simulink model "gm_DUALportRAMinterface_v3_vnl"  (R2024a)
settings: Solver=FixedStepDiscrete  StartTime=0.0  StopTime=20  RelTol=1e-3
undefined symbols (not defined in the file or in its folder): magnitude, Ts
libraries: hdlsllib x419, hdlmdlgenlib x103, embmathops x12, simulink x5, dsphdlxfrm2 x2
(part 7 of 11)

== system gm_DUALportRAMinterface_v3_vnl/PL/integration_block1/GA_main/coefficent_array/individual4 ==
  reg_in : Inport  OutDataTypeStr=fixdt(1, 33, 15)  PortDimensions=1  SampleTime=3.00000003e-08
  reg_in1 : Inport  Port=2  OutDataTypeStr=fixdt(1, 33, 15)  PortDimensions=1  SampleTime=3.00000003e-08
  reg_in2 : Inport  Port=3  OutDataTypeStr=fixdt(1, 33, 15)  PortDimensions=1  SampleTime=3.00000003e-08
  reg_in3 : Inport  Port=4  OutDataTypeStr=fixdt(1, 33, 15)  PortDimensions=1  SampleTime=3.00000003e-08
  reg_in4 : Inport  Port=5  OutDataTypeStr=fixdt(1, 33, 15)  PortDimensions=1  SampleTime=3.00000003e-08
  reg_in5 : Inport  Port=6  OutDataTypeStr=fixdt(1, 33, 15)  PortDimensions=1  SampleTime=3.00000003e-08
  reg_in6 : Inport  Port=7  OutDataTypeStr=fixdt(1, 33, 15)  PortDimensions=1  SampleTime=3.00000003e-08
  enable : Inport  Port=8  OutDataTypeStr=boolean  PortDimensions=1  SampleTime=3.00000003e-08
  Subsystem : Subsystem
  Subsystem1 : Subsystem
  Subsystem2 : Subsystem
  Subsystem3 : Subsystem
  Subsystem4 : Subsystem
  Subsystem5 : Subsystem
  Subsystem6 : Subsystem
  score : Outport  SampleTime=3.00000003e-08
  a2 : Outport  Port=2  SampleTime=3.00000003e-08
  a3 : Outport  Port=3  SampleTime=3.00000003e-08
  a4 : Outport  Port=4  SampleTime=3.00000003e-08
  b2 : Outport  Port=5  SampleTime=3.00000003e-08
  b3 : Outport  Port=6  SampleTime=3.00000003e-08
  b4 : Outport  Port=7  SampleTime=3.00000003e-08
  wires:
  Subsystem6/1(reg_out) -> b4/1
  Subsystem5/1(reg_out) -> b3/1
  Subsystem4/1(reg_out) -> b2/1
  Subsystem3/1(reg_out) -> a4/1
  Subsystem2/1(reg_out) -> a3/1
  Subsystem1/1(reg_out) -> a2/1
  Subsystem/1(reg_out) -> score/1
  enable/1 -> Subsystem3/2(enable), Subsystem4/2(enable), Subsystem5/2(enable), Subsystem6/2(enable), Subsystem2/2(enable), Subsystem1/2(enable), Subsystem/2(enable)
  reg_in6/1 -> Subsystem6/1(reg_in)
  reg_in5/1 -> Subsystem5/1(reg_in)
  reg_in4/1 -> Subsystem4/1(reg_in)
  reg_in3/1 -> Subsystem3/1(reg_in)
  reg_in2/1 -> Subsystem2/1(reg_in)
  reg_in1/1 -> Subsystem1/1(reg_in)
  reg_in/1 -> Subsystem/1(reg_in)

== system gm_DUALportRAMinterface_v3_vnl/PL/integration_block1/GA_main/coefficent_array/output_selector ==
  chose_port : Inport  OutDataTypeStr=fixdt(0, 4, 0)  PortDimensions=1  SampleTime=3.00000003e-08
  In2 : Inport  Port=2  OutDataTypeStr=fixdt(1, 33, 15)  PortDimensions=[7]  SampleTime=3.00000003e-08
  In3 : Inport  Port=3  OutDataTypeStr=fixdt(1, 33, 15)  PortDimensions=[7]  SampleTime=3.00000003e-08
  In4 : Inport  Port=4  OutDataTypeStr=fixdt(1, 33, 15)  PortDimensions=[7]  SampleTime=3.00000003e-08
  In5 : Inport  Port=5  OutDataTypeStr=fixdt(1, 33, 15)  PortDimensions=[7]  SampleTime=3.00000003e-08
  Multiport Switch : MultiPortSwitch  Inputs=4  OutDataTypeStr=fixdt(1, 33, 15)  SaturateOnIntegerOverflow=off  InputSameDT=off
  Switch : Switch  Criteria=u2 > Threshold  OutDataTypeStr=fixdt(1, 33, 15)  SaturateOnIntegerOverflow=off  InputSameDT=off
  Switch1 : Switch  Criteria=u2 > Threshold  OutDataTypeStr=fixdt(0, 4, 0)  SaturateOnIntegerOverflow=off  InputSameDT=off
  default_value : Constant  OutDataTypeStr=fixdt(0,4,0)  SampleTime=Ts
  ensure_correct_output : Constant  Value=0  OutDataTypeStr=fixdt(0,1,0)  SampleTime=Ts
  Out1 : Outport  SampleTime=3.00000003e-08
  wires:
  ensure_correct_output/1 -> Switch/3
  default_value/1 -> Switch1/3
  Switch1/1 -> Multiport Switch/1
  Switch/1 -> Out1/1
  Multiport Switch/1 -> Switch/1
  In5/1 -> Multiport Switch/5
  In4/1 -> Multiport Switch/4
  In3/1 -> Multiport Switch/3
  In2/1 -> Multiport Switch/2
  chose_port/1 -> Switch/2, Switch1/1, Switch1/2

== system gm_DUALportRAMinterface_v3_vnl/PL/integration_block1/GA_main/coefficent_array/swap_counter ==
  In1 : Inport  OutDataTypeStr=boolean  PortDimensions=1  SampleTime=3.00000003e-08
  In2 : Inport  Port=2  OutDataTypeStr=boolean  PortDimensions=1  SampleTime=3.00000003e-08
  Add : Sum  OutDataTypeStr=fixdt(0,4,0)  AccumDataTypeStr=fixdt(0,4,0)
  Constant18 : Constant  OutDataTypeStr=fixdt(0,4,0)  SampleTime=Ts
  Constant19 : Constant  Value=0  OutDataTypeStr=fixdt(0,4,0)  SampleTime=Ts
  Constant20 : Constant  Value=0  OutDataTypeStr=fixdt(0,4,0)  SampleTime=Ts
  Delay : Delay  DelayLength=1  InitialCondition=0  SampleTime=Ts
  Switch : Switch  Criteria=u2 > Threshold  OutDataTypeStr=fixdt(0,4,0)  SaturateOnIntegerOverflow=off  InputSameDT=off
  Switch8 : Switch  Criteria=u2 > Threshold  OutDataTypeStr=fixdt(0,4,0)  SaturateOnIntegerOverflow=off  InputSameDT=off
  Out1 : Outport  SampleTime=3.00000003e-08
  wires:
  Switch8/1 -> Add/2
  Add/1 -> Delay/1
  Switch/1 -> Add/1
  In2/1 -> Switch8/2
  Constant20/1 -> Switch8/1
  Delay/1 -> Switch8/3, Out1/1
  Constant19/1 -> Switch/3
  Constant18/1 -> Switch/1
  In1/1 -> Switch/2

== system gm_DUALportRAMinterface_v3_vnl/PL/integration_block1/GA_main/coefficent_array/swap_counter1 ==
  In1 : Inport  OutDataTypeStr=boolean  PortDimensions=1  SampleTime=3.00000003e-08
  In2 : Inport  Port=2  OutDataTypeStr=boolean  PortDimensions=1  SampleTime=3.00000003e-08
  Add : Sum  OutDataTypeStr=fixdt(0,4,0)  AccumDataTypeStr=fixdt(0,4,0)
  Constant18 : Constant  OutDataTypeStr=fixdt(0,4,0)  SampleTime=Ts
  Constant19 : Constant  Value=0  OutDataTypeStr=fixdt(0,4,0)  SampleTime=Ts
  Constant20 : Constant  OutDataTypeStr=fixdt(0,4,0)  SampleTime=Ts
  Delay : Delay  DelayLength=1  InitialCondition=0  SampleTime=Ts
  Switch : Switch  Criteria=u2 > Threshold  OutDataTypeStr=fixdt(0,4,0)  SaturateOnIntegerOverflow=off  InputSameDT=off
  Switch8 : Switch  Criteria=u2 > Threshold  OutDataTypeStr=fixdt(0,4,0)  SaturateOnIntegerOverflow=off  InputSameDT=off
  Out1 : Outport  SampleTime=3.00000003e-08
  wires:
  Switch8/1 -> Add/2
  Add/1 -> Delay/1
  Switch/1 -> Add/1
  In2/1 -> Switch8/2
  Constant20/1 -> Switch8/1
  Delay/1 -> Switch8/3, Out1/1
  Constant19/1 -> Switch/3
  Constant18/1 -> Switch/1
  In1/1 -> Switch/2

== system gm_DUALportRAMinterface_v3_vnl/PL/integration_block1/GA_main/coefficent_array1/Chart ==
  index : Inport  OutDataTypeStr=fixdt(0, 4, 0)  PortDimensions=1  SampleTime=3.00000003e-08
  start_sort : Inport  Port=2  OutDataTypeStr=boolean  PortDimensions=1  SampleTime=3.00000003e-08
  swaps_in : Inport  Port=3  OutDataTypeStr=fixdt(0, 4, 0)  PortDimensions=1  SampleTime=3.00000003e-08
  swap_signal : Inport  Port=4  OutDataTypeStr=boolean  PortDimensions=1  SampleTime=3.00000003e-08
  Chart : Stateflow chart  TreatAsAtomicUnit=on
      settings: PortSchema="{\"entries\":[{\"content\":{\"sides\":[{\"content\":{\"connectorIds\":[\"In1\",\"In4\",\"In3\"]},\"type\":\"ConnectorPlacement.EquallySpacedRectSide\",\"uuid\":\"bd2dafac-a5a9-4836-b8bd-cefb36fb6626\"},{\"content\":{\"connectorIds\":[\"Out1\",\"Out2\",\"Out3\",\"Out4\",\"Out5\",\"Out6\"],\"side\":\"RIGHT\"},\"type\":\"ConnectorPlacement.EquallySpacedRectSide\",\"uuid\":\"b2eb894e-8d56-4038-acbe-51c43d919a15\"},{\"content\":{\"connectorIds\":[\"In2\"],\"side\":\"TOP\"},\"type\":\"ConnectorPlacement.EquallySpacedRectSide\",\"uuid\":\"645ecb99-1eca-4a2d-8e44-d34ac75e3d1a\"}]},\"type\":\"ConnectorPlacement.EquallySpacedConnector\",\"uuid\":\"63f53eab-c5ec-482c-b992-d953653b0c27\"}],\"packageUris\":[\"http://schema.mathworks.com/mf0/Connector/R2020b\"],\"version\":\"1.0\"}"
  index_increment : Outport  SampleTime=3.00000003e-08
  index_reset : Outport  Port=2  SampleTime=3.00000003e-08
  sort_done : Outport  Port=3  SampleTime=3.00000003e-08
  commit_swap : Outport  Port=4  SampleTime=3.00000003e-08
  swaps_increment : Outport  Port=5  SampleTime=3.00000003e-08
  reset_swaps : Outport  Port=6  SampleTime=3.00000003e-08
  wires:
  Chart/6(reset_swaps) -> reset_swaps/1
  Chart/5(swaps_increment) -> swaps_increment/1
  Chart/4(commit_swap) -> commit_swap/1
  Chart/3(sort_done) -> sort_done/1
  Chart/2(index_reset) -> index_reset/1
  Chart/1(index_increment) -> index_increment/1
  swap_signal/1 -> Chart/4(swap_signal)
  swaps_in/1 -> Chart/3(swaps_in)
  start_sort/1 -> Chart/2(start_sort)
  index/1 -> Chart/1(index)

== system gm_DUALportRAMinterface_v3_vnl/PL/integration_block1/GA_main/coefficent_array1/individual1 ==
  reg_in : Inport  OutDataTypeStr=fixdt(1, 33, 15)  PortDimensions=1  SampleTime=3.00000003e-08
  reg_in1 : Inport  Port=2  OutDataTypeStr=fixdt(1, 33, 15)  PortDimensions=1  SampleTime=3.00000003e-08
  reg_in2 : Inport  Port=3  OutDataTypeStr=fixdt(1, 33, 15)  PortDimensions=1  SampleTime=3.00000003e-08
  reg_in3 : Inport  Port=4  OutDataTypeStr=fixdt(1, 33, 15)  PortDimensions=1  SampleTime=3.00000003e-08
  reg_in4 : Inport  Port=5  OutDataTypeStr=fixdt(1, 33, 15)  PortDimensions=1  SampleTime=3.00000003e-08
  reg_in5 : Inport  Port=6  OutDataTypeStr=fixdt(1, 33, 15)  PortDimensions=1  SampleTime=3.00000003e-08
  reg_in6 : Inport  Port=7  OutDataTypeStr=fixdt(1, 33, 15)  PortDimensions=1  SampleTime=3.00000003e-08
  enable : Inport  Port=8  OutDataTypeStr=boolean  PortDimensions=1  SampleTime=3.00000003e-08
  Subsystem : Subsystem
  Subsystem1 : Subsystem
  Subsystem2 : Subsystem
  Subsystem3 : Subsystem
  Subsystem4 : Subsystem
  Subsystem5 : Subsystem
  Subsystem6 : Subsystem
  score : Outport  SampleTime=3.00000003e-08
  a2 : Outport  Port=2  SampleTime=3.00000003e-08
  a3 : Outport  Port=3  SampleTime=3.00000003e-08
  a4 : Outport  Port=4  SampleTime=3.00000003e-08
  b2 : Outport  Port=5  SampleTime=3.00000003e-08
  b3 : Outport  Port=6  SampleTime=3.00000003e-08
  b4 : Outport  Port=7  SampleTime=3.00000003e-08
  wires:
  Subsystem6/1(reg_out) -> b4/1
  Subsystem5/1(reg_out) -> b3/1
  Subsystem4/1(reg_out) -> b2/1
  Subsystem3/1(reg_out) -> a4/1
  Subsystem2/1(reg_out) -> a3/1
  Subsystem1/1(reg_out) -> a2/1
  Subsystem/1(reg_out) -> score/1
  enable/1 -> Subsystem3/2(enable), Subsystem4/2(enable), Subsystem5/2(enable), Subsystem6/2(enable), Subsystem2/2(enable), Subsystem1/2(enable), Subsystem/2(enable)
  reg_in6/1 -> Subsystem6/1(reg_in)
  reg_in5/1 -> Subsystem5/1(reg_in)
  reg_in4/1 -> Subsystem4/1(reg_in)
  reg_in3/1 -> Subsystem3/1(reg_in)
  reg_in2/1 -> Subsystem2/1(reg_in)
  reg_in1/1 -> Subsystem1/1(reg_in)
  reg_in/1 -> Subsystem/1(reg_in)

== system gm_DUALportRAMinterface_v3_vnl/PL/integration_block1/GA_main/coefficent_array1/individual2 ==
  reg_in : Inport  OutDataTypeStr=fixdt(1, 33, 15)  PortDimensions=1  SampleTime=3.00000003e-08
  reg_in1 : Inport  Port=2  OutDataTypeStr=fixdt(1, 33, 15)  PortDimensions=1  SampleTime=3.00000003e-08
  reg_in2 : Inport  Port=3  OutDataTypeStr=fixdt(1, 33, 15)  PortDimensions=1  SampleTime=3.00000003e-08
  reg_in3 : Inport  Port=4  OutDataTypeStr=fixdt(1, 33, 15)  PortDimensions=1  SampleTime=3.00000003e-08
  reg_in4 : Inport  Port=5  OutDataTypeStr=fixdt(1, 33, 15)  PortDimensions=1  SampleTime=3.00000003e-08
  reg_in5 : Inport  Port=6  OutDataTypeStr=fixdt(1, 33, 15)  PortDimensions=1  SampleTime=3.00000003e-08
  reg_in6 : Inport  Port=7  OutDataTypeStr=fixdt(1, 33, 15)  PortDimensions=1  SampleTime=3.00000003e-08
  enable : Inport  Port=8  OutDataTypeStr=boolean  PortDimensions=1  SampleTime=3.00000003e-08
  Subsystem : Subsystem
  Subsystem1 : Subsystem
  Subsystem2 : Subsystem
  Subsystem3 : Subsystem
  Subsystem4 : Subsystem
  Subsystem5 : Subsystem
  Subsystem6 : Subsystem
  score : Outport  SampleTime=3.00000003e-08
  a2 : Outport  Port=2  SampleTime=3.00000003e-08
  a3 : Outport  Port=3  SampleTime=3.00000003e-08
  a4 : Outport  Port=4  SampleTime=3.00000003e-08
  b2 : Outport  Port=5  SampleTime=3.00000003e-08
  b3 : Outport  Port=6  SampleTime=3.00000003e-08
  b4 : Outport  Port=7  SampleTime=3.00000003e-08
  wires:
  Subsystem6/1(reg_out) -> b4/1
  Subsystem5/1(reg_out) -> b3/1
  Subsystem4/1(reg_out) -> b2/1
  Subsystem3/1(reg_out) -> a4/1
  Subsystem2/1(reg_out) -> a3/1
  Subsystem1/1(reg_out) -> a2/1
  Subsystem/1(reg_out) -> score/1
  enable/1 -> Subsystem/2(enable), Subsystem1/2(enable), Subsystem2/2(enable), Subsystem6/2(enable), Subsystem5/2(enable), Subsystem4/2(enable), Subsystem3/2(enable)
  reg_in6/1 -> Subsystem6/1(reg_in)
  reg_in5/1 -> Subsystem5/1(reg_in)
  reg_in4/1 -> Subsystem4/1(reg_in)
  reg_in3/1 -> Subsystem3/1(reg_in)
  reg_in2/1 -> Subsystem2/1(reg_in)
  reg_in1/1 -> Subsystem1/1(reg_in)
  reg_in/1 -> Subsystem/1(reg_in)

== system gm_DUALportRAMinterface_v3_vnl/PL/integration_block1/GA_main/coefficent_array1/individual3 ==
  reg_in : Inport  OutDataTypeStr=fixdt(1, 33, 15)  PortDimensions=1  SampleTime=3.00000003e-08
  reg_in1 : Inport  Port=2  OutDataTypeStr=fixdt(1, 33, 15)  PortDimensions=1  SampleTime=3.00000003e-08
  reg_in2 : Inport  Port=3  OutDataTypeStr=fixdt(1, 33, 15)  PortDimensions=1  SampleTime=3.00000003e-08
  reg_in3 : Inport  Port=4  OutDataTypeStr=fixdt(1, 33, 15)  PortDimensions=1  SampleTime=3.00000003e-08
  reg_in4 : Inport  Port=5  OutDataTypeStr=fixdt(1, 33, 15)  PortDimensions=1  SampleTime=3.00000003e-08
  reg_in5 : Inport  Port=6  OutDataTypeStr=fixdt(1, 33, 15)  PortDimensions=1  SampleTime=3.00000003e-08
  reg_in6 : Inport  Port=7  OutDataTypeStr=fixdt(1, 33, 15)  PortDimensions=1  SampleTime=3.00000003e-08
  enable : Inport  Port=8  OutDataTypeStr=boolean  PortDimensions=1  SampleTime=3.00000003e-08
  Subsystem : Subsystem
  Subsystem1 : Subsystem
  Subsystem2 : Subsystem
  Subsystem3 : Subsystem
  Subsystem4 : Subsystem
  Subsystem5 : Subsystem
  Subsystem6 : Subsystem
  score : Outport  SampleTime=3.00000003e-08
  a2 : Outport  Port=2  SampleTime=3.00000003e-08
  a3 : Outport  Port=3  SampleTime=3.00000003e-08
  a4 : Outport  Port=4  SampleTime=3.00000003e-08
  b2 : Outport  Port=5  SampleTime=3.00000003e-08
  b3 : Outport  Port=6  SampleTime=3.00000003e-08
  b4 : Outport  Port=7  SampleTime=3.00000003e-08
  wires:
  Subsystem6/1(reg_out) -> b4/1
  Subsystem5/1(reg_out) -> b3/1
  Subsystem4/1(reg_out) -> b2/1
  Subsystem3/1(reg_out) -> a4/1
  Subsystem2/1(reg_out) -> a3/1
  Subsystem1/1(reg_out) -> a2/1
  Subsystem/1(reg_out) -> score/1
  enable/1 -> Subsystem3/2(enable), Subsystem4/2(enable), Subsystem5/2(enable), Subsystem6/2(enable), Subsystem2/2(enable), Subsystem1/2(enable), Subsystem/2(enable)
  reg_in6/1 -> Subsystem6/1(reg_in)
  reg_in5/1 -> Subsystem5/1(reg_in)
  reg_in4/1 -> Subsystem4/1(reg_in)
  reg_in3/1 -> Subsystem3/1(reg_in)
  reg_in2/1 -> Subsystem2/1(reg_in)
  reg_in1/1 -> Subsystem1/1(reg_in)
  reg_in/1 -> Subsystem/1(reg_in)

== system gm_DUALportRAMinterface_v3_vnl/PL/integration_block1/GA_main/coefficent_array1/individual4 ==
  reg_in : Inport  OutDataTypeStr=fixdt(1, 33, 15)  PortDimensions=1  SampleTime=3.00000003e-08
  reg_in1 : Inport  Port=2  OutDataTypeStr=fixdt(1, 33, 15)  PortDimensions=1  SampleTime=3.00000003e-08
  reg_in2 : Inport  Port=3  OutDataTypeStr=fixdt(1, 33, 15)  PortDimensions=1  SampleTime=3.00000003e-08
  reg_in3 : Inport  Port=4  OutDataTypeStr=fixdt(1, 33, 15)  PortDimensions=1  SampleTime=3.00000003e-08
  reg_in4 : Inport  Port=5  OutDataTypeStr=fixdt(1, 33, 15)  PortDimensions=1  SampleTime=3.00000003e-08
  reg_in5 : Inport  Port=6  OutDataTypeStr=fixdt(1, 33, 15)  PortDimensions=1  SampleTime=3.00000003e-08
  reg_in6 : Inport  Port=7  OutDataTypeStr=fixdt(1, 33, 15)  PortDimensions=1  SampleTime=3.00000003e-08
  enable : Inport  Port=8  OutDataTypeStr=boolean  PortDimensions=1  SampleTime=3.00000003e-08
  Subsystem : Subsystem
  Subsystem1 : Subsystem
  Subsystem2 : Subsystem
  Subsystem3 : Subsystem
  Subsystem4 : Subsystem
  Subsystem5 : Subsystem
  Subsystem6 : Subsystem
  score : Outport  SampleTime=3.00000003e-08
  a2 : Outport  Port=2  SampleTime=3.00000003e-08
  a3 : Outport  Port=3  SampleTime=3.00000003e-08
  a4 : Outport  Port=4  SampleTime=3.00000003e-08
  b2 : Outport  Port=5  SampleTime=3.00000003e-08
  b3 : Outport  Port=6  SampleTime=3.00000003e-08
  b4 : Outport  Port=7  SampleTime=3.00000003e-08
  wires:
  Subsystem6/1(reg_out) -> b4/1
  Subsystem5/1(reg_out) -> b3/1
  Subsystem4/1(reg_out) -> b2/1
  Subsystem3/1(reg_out) -> a4/1
  Subsystem2/1(reg_out) -> a3/1
  Subsystem1/1(reg_out) -> a2/1
  Subsystem/1(reg_out) -> score/1
  enable/1 -> Subsystem/2(enable), Subsystem1/2(enable), Subsystem2/2(enable), Subsystem6/2(enable), Subsystem5/2(enable), Subsystem4/2(enable), Subsystem3/2(enable)
  reg_in6/1 -> Subsystem6/1(reg_in)
  reg_in5/1 -> Subsystem5/1(reg_in)
  reg_in4/1 -> Subsystem4/1(reg_in)
  reg_in3/1 -> Subsystem3/1(reg_in)
  reg_in2/1 -> Subsystem2/1(reg_in)
  reg_in1/1 -> Subsystem1/1(reg_in)
  reg_in/1 -> Subsystem/1(reg_in)

== system gm_DUALportRAMinterface_v3_vnl/PL/integration_block1/GA_main/coefficent_array1/output_selector ==
  chose_port : Inport  OutDataTypeStr=fixdt(0, 4, 0)  PortDimensions=1  SampleTime=3.00000003e-08
  In2 : Inport  Port=2  OutDataTypeStr=fixdt(1, 33, 15)  PortDimensions=[7]  SampleTime=3.00000003e-08
  In3 : Inport  Port=3  OutDataTypeStr=fixdt(1, 33, 15)  PortDimensions=[7]  SampleTime=3.00000003e-08
  In4 : Inport  Port=4  OutDataTypeStr=fixdt(1, 33, 15)  PortDimensions=[7]  SampleTime=3.00000003e-08
  In5 : Inport  Port=5  OutDataTypeStr=fixdt(1, 33, 15)  PortDimensions=[7]  SampleTime=3.00000003e-08
  Multiport Switch : MultiPortSwitch  Inputs=4  OutDataTypeStr=fixdt(1, 33, 15)  SaturateOnIntegerOverflow=off  InputSameDT=off
  Switch : Switch  Criteria=u2 > Threshold  OutDataTypeStr=fixdt(1, 33, 15)  SaturateOnIntegerOverflow=off  InputSameDT=off
  Switch1 : Switch  Criteria=u2 > Threshold  OutDataTypeStr=fixdt(0, 4, 0)  SaturateOnIntegerOverflow=off  InputSameDT=off
  default_value : Constant  OutDataTypeStr=fixdt(0,4,0)  SampleTime=Ts
  ensure_correct_output : Constant  Value=0  OutDataTypeStr=fixdt(0,1,0)  SampleTime=Ts
  Out1 : Outport  SampleTime=3.00000003e-08
  wires:
  ensure_correct_output/1 -> Switch/3
  default_value/1 -> Switch1/3
  Switch1/1 -> Multiport Switch/1
  Switch/1 -> Out1/1
  Multiport Switch/1 -> Switch/1
  In5/1 -> Multiport Switch/5
  In4/1 -> Multiport Switch/4
  In3/1 -> Multiport Switch/3
  In2/1 -> Multiport Switch/2
  chose_port/1 -> Switch/2, Switch1/1, Switch1/2

== system gm_DUALportRAMinterface_v3_vnl/PL/integration_block1/GA_main/coefficent_array1/swap_counter ==
  In1 : Inport  OutDataTypeStr=boolean  PortDimensions=1  SampleTime=3.00000003e-08
  In2 : Inport  Port=2  OutDataTypeStr=boolean  PortDimensions=1  SampleTime=3.00000003e-08
  Add : Sum  OutDataTypeStr=fixdt(0,4,0)  AccumDataTypeStr=fixdt(0,4,0)
  Constant18 : Constant  OutDataTypeStr=fixdt(0,4,0)  SampleTime=Ts
  Constant19 : Constant  Value=0  OutDataTypeStr=fixdt(0,4,0)  SampleTime=Ts
  Constant20 : Constant  Value=0  OutDataTypeStr=fixdt(0,4,0)  SampleTime=Ts
  Delay : Delay  DelayLength=1  InitialCondition=0  SampleTime=Ts
  Switch : Switch  Criteria=u2 > Threshold  OutDataTypeStr=fixdt(0,4,0)  SaturateOnIntegerOverflow=off  InputSameDT=off
  Switch8 : Switch  Criteria=u2 > Threshold  OutDataTypeStr=fixdt(0,4,0)  SaturateOnIntegerOverflow=off  InputSameDT=off
  Out1 : Outport  SampleTime=3.00000003e-08
  wires:
  Switch8/1 -> Add/2
  Add/1 -> Delay/1
  Switch/1 -> Add/1
  In2/1 -> Switch8/2
  Constant20/1 -> Switch8/1
  Delay/1 -> Switch8/3, Out1/1
  Constant19/1 -> Switch/3
  Constant18/1 -> Switch/1
  In1/1 -> Switch/2

== system gm_DUALportRAMinterface_v3_vnl/PL/integration_block1/GA_main/coefficent_array1/swap_counter1 ==
  In1 : Inport  OutDataTypeStr=boolean  PortDimensions=1  SampleTime=3.00000003e-08
  In2 : Inport  Port=2  OutDataTypeStr=boolean  PortDimensions=1  SampleTime=3.00000003e-08
  Add : Sum  OutDataTypeStr=fixdt(0,4,0)  AccumDataTypeStr=fixdt(0,4,0)
  Constant18 : Constant  OutDataTypeStr=fixdt(0,4,0)  SampleTime=Ts
  Constant19 : Constant  Value=0  OutDataTypeStr=fixdt(0,4,0)  SampleTime=Ts
  Constant20 : Constant  OutDataTypeStr=fixdt(0,4,0)  SampleTime=Ts
  Delay : Delay  DelayLength=1  InitialCondition=0  SampleTime=Ts
  Switch : Switch  Criteria=u2 > Threshold  OutDataTypeStr=fixdt(0,4,0)  SaturateOnIntegerOverflow=off  InputSameDT=off
  Switch8 : Switch  Criteria=u2 > Threshold  OutDataTypeStr=fixdt(0,4,0)  SaturateOnIntegerOverflow=off  InputSameDT=off
  Out1 : Outport  SampleTime=3.00000003e-08
  wires:
  Switch8/1 -> Add/2
  Add/1 -> Delay/1
  Switch/1 -> Add/1
  In2/1 -> Switch8/2
  Constant20/1 -> Switch8/1
  Delay/1 -> Switch8/3, Out1/1
  Constant19/1 -> Switch/3
  Constant18/1 -> Switch/1
  In1/1 -> Switch/2

== system gm_DUALportRAMinterface_v3_vnl/PL/integration_block1/Subsystem/16bLFSR/10 ==
  reg_in : Inport  OutDataTypeStr=boolean  PortDimensions=1  SampleTime=3.00000003e-08
  Delay : Delay  DelayLength=1  InitialCondition=0  SampleTime=Ts
  reg_out : Outport  SampleTime=3.00000003e-08
  wires:
  Delay/1 -> reg_out/1
  reg_in/1 -> Delay/1

== system gm_DUALportRAMinterface_v3_vnl/PL/integration_block1/Subsystem/16bLFSR/11 ==
  reg_in : Inport  OutDataTypeStr=boolean  PortDimensions=1  SampleTime=3.00000003e-08
  Delay : Delay  DelayLength=1  InitialCondition=0  SampleTime=Ts
  reg_out : Outport  SampleTime=3.00000003e-08
  wires:
  Delay/1 -> reg_out/1
  reg_in/1 -> Delay/1

== system gm_DUALportRAMinterface_v3_vnl/PL/integration_block1/Subsystem/16bLFSR/12 ==
  reg_in : Inport  OutDataTypeStr=boolean  PortDimensions=1  SampleTime=3.00000003e-08
  Delay : Delay  DelayLength=1  InitialCondition=0  SampleTime=Ts
  reg_out : Outport  SampleTime=3.00000003e-08
  wires:
  Delay/1 -> reg_out/1
  reg_in/1 -> Delay/1

== system gm_DUALportRAMinterface_v3_vnl/PL/integration_block1/Subsystem/16bLFSR/13 ==
  reg_in : Inport  OutDataTypeStr=boolean  PortDimensions=1  SampleTime=3.00000003e-08
  Delay : Delay  DelayLength=1  InitialCondition=0  SampleTime=Ts
  reg_out : Outport  SampleTime=3.00000003e-08
  wires:
  Delay/1 -> reg_out/1
  reg_in/1 -> Delay/1

== system gm_DUALportRAMinterface_v3_vnl/PL/integration_block1/Subsystem/16bLFSR/14 ==
  reg_in : Inport  OutDataTypeStr=boolean  PortDimensions=1  SampleTime=3.00000003e-08
  Delay : Delay  DelayLength=1  InitialCondition=0  SampleTime=Ts
  reg_out : Outport  SampleTime=3.00000003e-08
  wires:
  Delay/1 -> reg_out/1
  reg_in/1 -> Delay/1

== system gm_DUALportRAMinterface_v3_vnl/PL/integration_block1/Subsystem/16bLFSR/15 ==
  reg_in : Inport  OutDataTypeStr=boolean  PortDimensions=1  SampleTime=3.00000003e-08
  Delay : Delay  DelayLength=1  InitialCondition=0  SampleTime=Ts
  reg_out : Outport  SampleTime=3.00000003e-08
  wires:
  Delay/1 -> reg_out/1
  reg_in/1 -> Delay/1

== system gm_DUALportRAMinterface_v3_vnl/PL/integration_block1/Subsystem/16bLFSR/16 ==
  reg_in : Inport  OutDataTypeStr=boolean  PortDimensions=1  SampleTime=3.00000003e-08
  Delay : Delay  DelayLength=1  InitialCondition=0  SampleTime=Ts
  reg_out : Outport  SampleTime=3.00000003e-08
  wires:
  Delay/1 -> reg_out/1
  reg_in/1 -> Delay/1

== system gm_DUALportRAMinterface_v3_vnl/PL/integration_block1/Subsystem/16bLFSR/1_ss ==
  reg_in : Inport  OutDataTypeStr=boolean  PortDimensions=1  SampleTime=3.00000003e-08
  Delay : Delay  DelayLength=1  InitialCondition=0  SampleTime=Ts
  reg_out : Outport  SampleTime=3.00000003e-08
  wires:
  Delay/1 -> reg_out/1
  reg_in/1 -> Delay/1

== system gm_DUALportRAMinterface_v3_vnl/PL/integration_block1/Subsystem/16bLFSR/2_ss ==
  reg_in : Inport  OutDataTypeStr=boolean  PortDimensions=1  SampleTime=3.00000003e-08
  Delay : Delay  DelayLength=1  InitialCondition=0  SampleTime=Ts
  reg_out : Outport  SampleTime=3.00000003e-08
  wires:
  Delay/1 -> reg_out/1
  reg_in/1 -> Delay/1

== system gm_DUALportRAMinterface_v3_vnl/PL/integration_block1/Subsystem/16bLFSR/3_ss ==
  reg_in : Inport  OutDataTypeStr=boolean  PortDimensions=1  SampleTime=3.00000003e-08
  Delay : Delay  DelayLength=1  InitialCondition=0  SampleTime=Ts
  reg_out : Outport  SampleTime=3.00000003e-08
  wires:
  Delay/1 -> reg_out/1
  reg_in/1 -> Delay/1

== system gm_DUALportRAMinterface_v3_vnl/PL/integration_block1/Subsystem/16bLFSR/4_ss ==
  reg_in : Inport  OutDataTypeStr=boolean  PortDimensions=1  SampleTime=3.00000003e-08
  Delay : Delay  DelayLength=1  InitialCondition=0  SampleTime=Ts
  reg_out : Outport  SampleTime=3.00000003e-08
  wires:
  Delay/1 -> reg_out/1
  reg_in/1 -> Delay/1

== system gm_DUALportRAMinterface_v3_vnl/PL/integration_block1/Subsystem/16bLFSR/5_ss ==
  reg_in : Inport  OutDataTypeStr=boolean  PortDimensions=1  SampleTime=3.00000003e-08
  Delay : Delay  DelayLength=1  InitialCondition=0  SampleTime=Ts
  reg_out : Outport  SampleTime=3.00000003e-08
  wires:
  Delay/1 -> reg_out/1
  reg_in/1 -> Delay/1

== system gm_DUALportRAMinterface_v3_vnl/PL/integration_block1/Subsystem/16bLFSR/6_ss ==
  reg_in : Inport  OutDataTypeStr=boolean  PortDimensions=1  SampleTime=3.00000003e-08
  Delay : Delay  DelayLength=1  InitialCondition=0  SampleTime=Ts
  reg_out : Outport  SampleTime=3.00000003e-08
  wires:
  Delay/1 -> reg_out/1
  reg_in/1 -> Delay/1

== system gm_DUALportRAMinterface_v3_vnl/PL/integration_block1/Subsystem/16bLFSR/7_ss ==
  reg_in : Inport  OutDataTypeStr=boolean  PortDimensions=1  SampleTime=3.00000003e-08
  Delay : Delay  DelayLength=1  InitialCondition=0  SampleTime=Ts
  reg_out : Outport  SampleTime=3.00000003e-08
  wires:
  Delay/1 -> reg_out/1
  reg_in/1 -> Delay/1

== system gm_DUALportRAMinterface_v3_vnl/PL/integration_block1/Subsystem/16bLFSR/8_ss ==
  reg_in : Inport  OutDataTypeStr=boolean  PortDimensions=1  SampleTime=3.00000003e-08
  Delay : Delay  DelayLength=1  InitialCondition=0  SampleTime=Ts
  reg_out : Outport  SampleTime=3.00000003e-08
  wires:
  Delay/1 -> reg_out/1
  reg_in/1 -> Delay/1

== system gm_DUALportRAMinterface_v3_vnl/PL/integration_block1/Subsystem/16bLFSR/9_ss ==
  reg_in : Inport  OutDataTypeStr=boolean  PortDimensions=1  SampleTime=3.00000003e-08
  Delay : Delay  DelayLength=1  InitialCondition=0  SampleTime=Ts
  reg_out : Outport  SampleTime=3.00000003e-08
  wires:
  Delay/1 -> reg_out/1
  reg_in/1 -> Delay/1

== system gm_DUALportRAMinterface_v3_vnl/PL/integration_block1/Subsystem/16bLFSR1/10 ==
  reg_in : Inport  OutDataTypeStr=boolean  PortDimensions=1  SampleTime=3.00000003e-08
  Delay : Delay  DelayLength=1  InitialCondition=0  SampleTime=Ts
  reg_out : Outport  SampleTime=3.00000003e-08
  wires:
  Delay/1 -> reg_out/1
  reg_in/1 -> Delay/1

== system gm_DUALportRAMinterface_v3_vnl/PL/integration_block1/Subsystem/16bLFSR1/11 ==
  reg_in : Inport  OutDataTypeStr=boolean  PortDimensions=1  SampleTime=3.00000003e-08
  Delay : Delay  DelayLength=1  InitialCondition=0  SampleTime=Ts
  reg_out : Outport  SampleTime=3.00000003e-08
  wires:
  Delay/1 -> reg_out/1
  reg_in/1 -> Delay/1

== system gm_DUALportRAMinterface_v3_vnl/PL/integration_block1/Subsystem/16bLFSR1/12 ==
  reg_in : Inport  OutDataTypeStr=boolean  PortDimensions=1  SampleTime=3.00000003e-08
  Delay : Delay  DelayLength=1  InitialCondition=0  SampleTime=Ts
  reg_out : Outport  SampleTime=3.00000003e-08
  wires:
  Delay/1 -> reg_out/1
  reg_in/1 -> Delay/1

== system gm_DUALportRAMinterface_v3_vnl/PL/integration_block1/Subsystem/16bLFSR1/13 ==
  reg_in : Inport  OutDataTypeStr=boolean  PortDimensions=1  SampleTime=3.00000003e-08
  Delay : Delay  DelayLength=1  InitialCondition=0  SampleTime=Ts
  reg_out : Outport  SampleTime=3.00000003e-08
  wires:
  Delay/1 -> reg_out/1
  reg_in/1 -> Delay/1

== system gm_DUALportRAMinterface_v3_vnl/PL/integration_block1/Subsystem/16bLFSR1/14 ==
  reg_in : Inport  OutDataTypeStr=boolean  PortDimensions=1  SampleTime=3.00000003e-08
  Delay : Delay  DelayLength=1  InitialCondition=0  SampleTime=Ts
  reg_out : Outport  SampleTime=3.00000003e-08
  wires:
  Delay/1 -> reg_out/1
  reg_in/1 -> Delay/1

== system gm_DUALportRAMinterface_v3_vnl/PL/integration_block1/Subsystem/16bLFSR1/15 ==
  reg_in : Inport  OutDataTypeStr=boolean  PortDimensions=1  SampleTime=3.00000003e-08
  Delay : Delay  DelayLength=1  InitialCondition=0  SampleTime=Ts
  reg_out : Outport  SampleTime=3.00000003e-08
  wires:
  Delay/1 -> reg_out/1
  reg_in/1 -> Delay/1

== system gm_DUALportRAMinterface_v3_vnl/PL/integration_block1/Subsystem/16bLFSR1/16 ==
  reg_in : Inport  OutDataTypeStr=boolean  PortDimensions=1  SampleTime=3.00000003e-08
  Delay : Delay  DelayLength=1  InitialCondition=0  SampleTime=Ts
  reg_out : Outport  SampleTime=3.00000003e-08
  wires:
  Delay/1 -> reg_out/1
  reg_in/1 -> Delay/1

== system gm_DUALportRAMinterface_v3_vnl/PL/integration_block1/Subsystem/16bLFSR1/1_ss ==
  reg_in : Inport  OutDataTypeStr=boolean  PortDimensions=1  SampleTime=3.00000003e-08
  Delay : Delay  DelayLength=1  InitialCondition=0  SampleTime=Ts
  reg_out : Outport  SampleTime=3.00000003e-08
  wires:
  Delay/1 -> reg_out/1
  reg_in/1 -> Delay/1

== system gm_DUALportRAMinterface_v3_vnl/PL/integration_block1/Subsystem/16bLFSR1/2_ss ==
  reg_in : Inport  OutDataTypeStr=boolean  PortDimensions=1  SampleTime=3.00000003e-08
  Delay : Delay  DelayLength=1  InitialCondition=0  SampleTime=Ts
  reg_out : Outport  SampleTime=3.00000003e-08
  wires:
  Delay/1 -> reg_out/1
  reg_in/1 -> Delay/1

== system gm_DUALportRAMinterface_v3_vnl/PL/integration_block1/Subsystem/16bLFSR1/3_ss ==
  reg_in : Inport  OutDataTypeStr=boolean  PortDimensions=1  SampleTime=3.00000003e-08
  Delay : Delay  DelayLength=1  InitialCondition=0  SampleTime=Ts
  reg_out : Outport  SampleTime=3.00000003e-08
  wires:
  Delay/1 -> reg_out/1
  reg_in/1 -> Delay/1

== system gm_DUALportRAMinterface_v3_vnl/PL/integration_block1/Subsystem/16bLFSR1/4_ss ==
  reg_in : Inport  OutDataTypeStr=boolean  PortDimensions=1  SampleTime=3.00000003e-08
  Delay : Delay  DelayLength=1  InitialCondition=0  SampleTime=Ts
  reg_out : Outport  SampleTime=3.00000003e-08
  wires:
  Delay/1 -> reg_out/1
  reg_in/1 -> Delay/1

== system gm_DUALportRAMinterface_v3_vnl/PL/integration_block1/Subsystem/16bLFSR1/5_ss ==
  reg_in : Inport  OutDataTypeStr=boolean  PortDimensions=1  SampleTime=3.00000003e-08
  Delay : Delay  DelayLength=1  InitialCondition=0  SampleTime=Ts
  reg_out : Outport  SampleTime=3.00000003e-08
  wires:
  Delay/1 -> reg_out/1
  reg_in/1 -> Delay/1

== system gm_DUALportRAMinterface_v3_vnl/PL/integration_block1/Subsystem/16bLFSR1/6_ss ==
  reg_in : Inport  OutDataTypeStr=boolean  PortDimensions=1  SampleTime=3.00000003e-08
  Delay : Delay  DelayLength=1  InitialCondition=0  SampleTime=Ts
  reg_out : Outport  SampleTime=3.00000003e-08
  wires:
  Delay/1 -> reg_out/1
  reg_in/1 -> Delay/1

== system gm_DUALportRAMinterface_v3_vnl/PL/integration_block1/Subsystem/16bLFSR1/7_ss ==
  reg_in : Inport  OutDataTypeStr=boolean  PortDimensions=1  SampleTime=3.00000003e-08
  Delay : Delay  DelayLength=1  InitialCondition=0  SampleTime=Ts
  reg_out : Outport  SampleTime=3.00000003e-08
  wires:
  Delay/1 -> reg_out/1
  reg_in/1 -> Delay/1

== system gm_DUALportRAMinterface_v3_vnl/PL/integration_block1/Subsystem/16bLFSR1/8_ss ==
  reg_in : Inport  OutDataTypeStr=boolean  PortDimensions=1  SampleTime=3.00000003e-08
  Delay : Delay  DelayLength=1  InitialCondition=0  SampleTime=Ts
  reg_out : Outport  SampleTime=3.00000003e-08
  wires:
  Delay/1 -> reg_out/1
  reg_in/1 -> Delay/1

== system gm_DUALportRAMinterface_v3_vnl/PL/integration_block1/Subsystem/16bLFSR1/9_ss ==
  reg_in : Inport  OutDataTypeStr=boolean  PortDimensions=1  SampleTime=3.00000003e-08
  Delay : Delay  DelayLength=1  InitialCondition=0  SampleTime=Ts
  reg_out : Outport  SampleTime=3.00000003e-08
  wires:
  Delay/1 -> reg_out/1
  reg_in/1 -> Delay/1

== system gm_DUALportRAMinterface_v3_vnl/PL/integration_block1/accumulator_scorer/64bitmsb_finder/8bit_PE1 ==
  D6 : Inport  OutDataTypeStr=fixdt(0, 1, 0)  PortDimensions=1  SampleTime=3.00000003e-08
  D5 : Inport  Port=2  OutDataTypeStr=fixdt(0, 1, 0)  PortDimensions=1  SampleTime=3.00000003e-08
  D4 : Inport  Port=3  OutDataTypeStr=fixdt(0, 1, 0)  PortDimensions=1  SampleTime=3.00000003e-08
  D3 : Inport  Port=4  OutDataTypeStr=fixdt(0, 1, 0)  PortDimensions=1  SampleTime=3.00000003e-08
  D2 : Inport  Port=5  OutDataTypeStr=fixdt(0, 1, 0)  PortDimensions=1  SampleTime=3.00000003e-08
  D1 : Inport  Port=6  OutDataTypeStr=fixdt(0, 1, 0)  PortDimensions=1  SampleTime=3.00000003e-08
  D0 : Inport  Port=7  OutDataTypeStr=fixdt(0, 1, 0)  PortDimensions=1  SampleTime=3.00000003e-08
  Add : Sum  OutDataTypeStr=fixdt(0, 5, 0)
  Bit Concat : hdlsllib/Logic and Bit Operations/Bit Concat  numInputs=3
  Constant : Constant  Value=0  OutDataTypeStr=boolean  SampleTime=Ts
  Constant2 : Constant  OutDataTypeStr=fixdt(0,4,0)  SampleTime=Ts
  Constant3 : Constant  Value=0  OutDataTypeStr=fixdt(0,4,0)  SampleTime=Ts
  Logical Operator{,10..16,22} (9 alike) : Logic  Operator=NOT  IconShape=distinctive  AllPortsSameDT=off  OutDataTypeStr=boolean
  Logical Operator1 : Logic  Operator=NAND  IconShape=distinctive  AllPortsSameDT=off  OutDataTypeStr=boolean
  Logical Operator{17..20} (4 alike) : Logic  Operator=OR  Inputs=4  IconShape=distinctive  AllPortsSameDT=off  OutDataTypeStr=boolean
  Logical Operator2 : Logic  Operator=NAND  Inputs=4  IconShape=distinctive  AllPortsSameDT=off  OutDataTypeStr=boolean
  Logical Operator21 : Logic  Operator=NAND  Inputs=3  IconShape=distinctive  AllPortsSameDT=off  OutDataTypeStr=boolean
  Logical Operator23 : Logic  IconShape=distinctive  AllPortsSameDT=off  OutDataTypeStr=boolean
  Logical Operator3 : Logic  Operator=NAND  Inputs=3  IconShape=distinctive  AllPortsSameDT=off  OutDataTypeStr=boolean
  Logical Operator4 : Logic  Inputs=3  IconShape=distinctive  AllPortsSameDT=off  OutDataTypeStr=boolean
  Logical Operator5 : Logic  Inputs=3  IconShape=distinctive  AllPortsSameDT=off  OutDataTypeStr=boolean
  Logical Operator6 : Logic  Inputs=4  IconShape=distinctive  AllPortsSameDT=off  OutDataTypeStr=boolean
  Logical Operator7 : Logic  Operator=NAND  Inputs=3  IconShape=distinctive  AllPortsSameDT=off  OutDataTypeStr=boolean
  Logical Operator8 : Logic  Operator=NAND  Inputs=4  IconShape=distinctive  AllPortsSameDT=off  OutDataTypeStr=boolean
  Logical Operator9 : Logic  Operator=NAND  Inputs=4  IconShape=distinctive  AllPortsSameDT=off  OutDataTypeStr=boolean
  Switch : Switch  Criteria=u2 > Threshold  OutDataTypeStr=fixdt(0, 4, 0)  SaturateOnIntegerOverflow=off  InputSameDT=off
  data2 : Outport  SampleTime=3.00000003e-08
  valid : Outport  Port=2  SampleTime=3.00000003e-08
  wires:
  Switch/1 -> Add/1
  Logical Operator9/1 -> Logical Operator16/1
  Logical Operator8/1 -> Logical Operator15/1, Logical Operator9/3
  Logical Operator7/1 -> Logical Operator14/1, Logical Operator8/3, Logical Operator9/2
  Logical Operator6/1 -> Logical Operator9/1
  Logical Operator5/1 -> Logical Operator8/1
  Logical Operator4/1 -> Logical Operator7/1
  Logical Operator3/1 -> Logical Operator12/1, Logical Operator2/1, Logical Operator4/1, Logical Operator5/1, Logical Operator6/1
  Logical Operator23/1 -> Switch/2
  Logical Operator22/1 -> Logical Operator23/2
  Logical Operator21/1 -> Logical Operator23/1
  Logical Operator20/1 -> valid/1, Logical Operator22/1
  Logical Operator2/1 -> Logical Operator13/1, Logical Operator6/4, Logical Operator7/2, Logical Operator8/2
  Logical Operator19/1 -> Bit Concat/3, Logical Operator20/4, Logical Operator21/3
  Logical Operator18/1 -> Bit Concat/2, Logical Operator20/3, Logical Operator21/2
  Logical Operator17/1 -> Bit Concat/1, Logical Operator20/1, Logical Operator21/1
  Logical Operator16/1 -> Logical Operator19/3
  Logical Operator15/1 -> Logical Operator18/4
  Logical Operator14/1 -> Logical Operator18/3, Logical Operator19/4
  Logical Operator13/1 -> Logical Operator17/4
  Logical Operator12/1 -> Logical Operator17/3, Logical Operator19/2
  Logical Operator11/1 -> Logical Operator17/2, Logical Operator18/2
  Logical Operator10/1 -> Logical Operator17/1, Logical Operator18/1, Logical Operator19/1
  Logical Operator1/1 -> Logical Operator11/1, Logical Operator2/2, Logical Operator3/1, Logical Operator4/2, Logical Operator5/2, Logical Operator6/2
  Logical Operator/1 -> Logical Operator1/1, Logical Operator10/1, Logical Operator2/3, Logical Operator3/2, Logical Operator4/3, Logical Operator5/3, Logical Operator6/3
  Constant3/1 -> Switch/1
  Constant2/1 -> Switch/3
  Constant/1 -> Logical Operator/1
  Bit Concat/1 -> Add/2
  Add/1 -> data2/1
  D0/1 -> Logical Operator20/2
  D1/1 -> Logical Operator9/4
  D2/1 -> Logical Operator8/4
  D3/1 -> Logical Operator7/3
  D4/1 -> Logical Operator2/4
  D5/1 -> Logical Operator3/3
  D6/1 -> Logical Operator1/2

== system gm_DUALportRAMinterface_v3_vnl/PL/integration_block1/accumulator_scorer/64bitmsb_finder/8bit_PE10 ==
  D7 : Inport  OutDataTypeStr=boolean  PortDimensions=1  SampleTime=3.00000003e-08
  D6 : Inport  Port=2  OutDataTypeStr=boolean  PortDimensions=1  SampleTime=3.00000003e-08
  D5 : Inport  Port=3  OutDataTypeStr=boolean  PortDimensions=1  SampleTime=3.00000003e-08
  D4 : Inport  Port=4  OutDataTypeStr=boolean  PortDimensions=1  SampleTime=3.00000003e-08
  D3 : Inport  Port=5  OutDataTypeStr=boolean  PortDimensions=1  SampleTime=3.00000003e-08
  D2 : Inport  Port=6  OutDataTypeStr=boolean  PortDimensions=1  SampleTime=3.00000003e-08
  D1 : Inport  Port=7  OutDataTypeStr=boolean  PortDimensions=1  SampleTime=3.00000003e-08
  D0 : Inport  Port=8  OutDataTypeStr=boolean  PortDimensions=1  SampleTime=3.00000003e-08
  Add : Sum  OutDataTypeStr=fixdt(0, 5, 0)
  Bit Concat : hdlsllib/Logic and Bit Operations/Bit Concat  numInputs=3
  Constant2 : Constant  OutDataTypeStr=fixdt(0,4,0)  SampleTime=Ts
  Constant3 : Constant  Value=0  OutDataTypeStr=fixdt(0,4,0)  SampleTime=Ts
  Logical Operator{,10..16,22} (9 alike) : Logic  Operator=NOT  IconShape=distinctive  AllPortsSameDT=off  OutDataTypeStr=boolean
  Logical Operator1 : Logic  Operator=NAND  IconShape=distinctive  AllPortsSameDT=off  OutDataTypeStr=boolean
  Logical Operator{17..20} (4 alike) : Logic  Operator=OR  Inputs=4  IconShape=distinctive  AllPortsSameDT=off  OutDataTypeStr=boolean
  Logical Operator2 : Logic  Operator=NAND  Inputs=4  IconShape=distinctive  AllPortsSameDT=off  OutDataTypeStr=boolean
  Logical Operator21 : Logic  Operator=NAND  Inputs=3  IconShape=distinctive  AllPortsSameDT=off  OutDataTypeStr=boolean
  Logical Operator23 : Logic  IconShape=distinctive  AllPortsSameDT=off  OutDataTypeStr=boolean
  Logical Operator3 : Logic  Operator=NAND  Inputs=3  IconShape=distinctive  AllPortsSameDT=off  OutDataTypeStr=boolean
  Logical Operator4 : Logic  Inputs=3  IconShape=distinctive  AllPortsSameDT=off  OutDataTypeStr=boolean
  Logical Operator5 : Logic  Inputs=3  IconShape=distinctive  AllPortsSameDT=off  OutDataTypeStr=boolean
  Logical Operator6 : Logic  Inputs=4  IconShape=distinctive  AllPortsSameDT=off  OutDataTypeStr=boolean
  Logical Operator7 : Logic  Operator=NAND  Inputs=3  IconShape=distinctive  AllPortsSameDT=off  OutDataTypeStr=boolean
  Logical Operator8 : Logic  Operator=NAND  Inputs=4  IconShape=distinctive  AllPortsSameDT=off  OutDataTypeStr=boolean
  Logical Operator9 : Logic  Operator=NAND  Inputs=4  IconShape=distinctive  AllPortsSameDT=off  OutDataTypeStr=boolean
  Switch : Switch  Criteria=u2 > Threshold  OutDataTypeStr=fixdt(0, 4, 0)  SaturateOnIntegerOverflow=off  InputSameDT=off
  data2 : Outport  SampleTime=3.00000003e-08
  valid : Outport  Port=2  SampleTime=3.00000003e-08
  wires:
  Switch/1 -> Add/1
  Logical Operator9/1 -> Logical Operator16/1
  Logical Operator8/1 -> Logical Operator15/1, Logical Operator9/3
  Logical Operator7/1 -> Logical Operator14/1, Logical Operator8/3, Logical Operator9/2
  Logical Operator6/1 -> Logical Operator9/1
  Logical Operator5/1 -> Logical Operator8/1
  Logical Operator4/1 -> Logical Operator7/1
  Logical Operator3/1 -> Logical Operator12/1, Logical Operator2/1, Logical Operator4/1, Logical Operator5/1, Logical Operator6/1
  Logical Operator23/1 -> Switch/2
  Logical Operator22/1 -> Logical Operator23/2
  Logical Operator21/1 -> Logical Operator23/1
  Logical Operator20/1 -> valid/1, Logical Operator22/1
  Logical Operator2/1 -> Logical Operator13/1, Logical Operator6/4, Logical Operator7/2, Logical Operator8/2
  Logical Operator19/1 -> Bit Concat/3, Logical Operator20/4, Logical Operator21/3
  Logical Operator18/1 -> Bit Concat/2, Logical Operator20/3, Logical Operator21/2
  Logical Operator17/1 -> Bit Concat/1, Logical Operator20/1, Logical Operator21/1
  Logical Operator16/1 -> Logical Operator19/3
  Logical Operator15/1 -> Logical Operator18/4
  Logical Operator14/1 -> Logical Operator18/3, Logical Operator19/4
  Logical Operator13/1 -> Logical Operator17/4
  Logical Operator12/1 -> Logical Operator17/3, Logical Operator19/2
  Logical Operator11/1 -> Logical Operator17/2, Logical Operator18/2
  Logical Operator10/1 -> Logical Operator17/1, Logical Operator18/1, Logical Operator19/1
  Logical Operator1/1 -> Logical Operator11/1, Logical Operator2/2, Logical Operator3/1, Logical Operator4/2, Logical Operator5/2, Logical Operator6/2
  Logical Operator/1 -> Logical Operator1/1, Logical Operator10/1, Logical Operator2/3, Logical Operator3/2, Logical Operator4/3, Logical Operator5/3, Logical Operator6/3
  Constant3/1 -> Switch/1
  Constant2/1 -> Switch/3
  Bit Concat/1 -> Add/2
  Add/1 -> data2/1
  D0/1 -> Logical Operator20/2
  D1/1 -> Logical Operator9/4
  D2/1 -> Logical Operator8/4
  D3/1 -> Logical Operator7/3
  D4/1 -> Logical Operator2/4
  D5/1 -> Logical Operator3/3
  D6/1 -> Logical Operator1/2
  D7/1 -> Logical Operator/1

== system gm_DUALportRAMinterface_v3_vnl/PL/integration_block1/accumulator_scorer/64bitmsb_finder/8bit_PE2 ==
  D7 : Inport  OutDataTypeStr=fixdt(0, 1, 0)  PortDimensions=1  SampleTime=3.00000003e-08
  D6 : Inport  Port=2  OutDataTypeStr=fixdt(0, 1, 0)  PortDimensions=1  SampleTime=3.00000003e-08
  D5 : Inport  Port=3  OutDataTypeStr=fixdt(0, 1, 0)  PortDimensions=1  SampleTime=3.00000003e-08
  D4 : Inport  Port=4  OutDataTypeStr=fixdt(0, 1, 0)  PortDimensions=1  SampleTime=3.00000003e-08
  D3 : Inport  Port=5  OutDataTypeStr=fixdt(0, 1, 0)  PortDimensions=1  SampleTime=3.00000003e-08
  D2 : Inport  Port=6  OutDataTypeStr=fixdt(0, 1, 0)  PortDimensions=1  SampleTime=3.00000003e-08
  D1 : Inport  Port=7  OutDataTypeStr=fixdt(0, 1, 0)  PortDimensions=1  SampleTime=3.00000003e-08
  D0 : Inport  Port=8  OutDataTypeStr=fixdt(0, 1, 0)  PortDimensions=1  SampleTime=3.00000003e-08
  Add : Sum  OutDataTypeStr=fixdt(0, 5, 0)
  Bit Concat : hdlsllib/Logic and Bit Operations/Bit Concat  numInputs=3
  Constant2 : Constant  OutDataTypeStr=fixdt(0,4,0)  SampleTime=Ts
  Constant3 : Constant  Value=0  OutDataTypeStr=fixdt(0,4,0)  SampleTime=Ts
  Logical Operator{,10..16,22} (9 alike) : Logic  Operator=NOT  IconShape=distinctive  AllPortsSameDT=off  OutDataTypeStr=boolean
  Logical Operator1 : Logic  Operator=NAND  IconShape=distinctive  AllPortsSameDT=off  OutDataTypeStr=boolean
  Logical Operator{17..20} (4 alike) : Logic  Operator=OR  Inputs=4  IconShape=distinctive  AllPortsSameDT=off  OutDataTypeStr=boolean
  Logical Operator2 : Logic  Operator=NAND  Inputs=4  IconShape=distinctive  AllPortsSameDT=off  OutDataTypeStr=boolean
  Logical Operator21 : Logic  Operator=NAND  Inputs=3  IconShape=distinctive  AllPortsSameDT=off  OutDataTypeStr=boolean
  Logical Operator23 : Logic  IconShape=distinctive  AllPortsSameDT=off  OutDataTypeStr=boolean
  Logical Operator3 : Logic  Operator=NAND  Inputs=3  IconShape=distinctive  AllPortsSameDT=off  OutDataTypeStr=boolean
  Logical Operator4 : Logic  Inputs=3  IconShape=distinctive  AllPortsSameDT=off  OutDataTypeStr=boolean
  Logical Operator5 : Logic  Inputs=3  IconShape=distinctive  AllPortsSameDT=off  OutDataTypeStr=boolean
  Logical Operator6 : Logic  Inputs=4  IconShape=distinctive  AllPortsSameDT=off  OutDataTypeStr=boolean
  Logical Operator7 : Logic  Operator=NAND  Inputs=3  IconShape=distinctive  AllPortsSameDT=off  OutDataTypeStr=boolean
  Logical Operator8 : Logic  Operator=NAND  Inputs=4  IconShape=distinctive  AllPortsSameDT=off  OutDataTypeStr=boolean
  Logical Operator9 : Logic  Operator=NAND  Inputs=4  IconShape=distinctive  AllPortsSameDT=off  OutDataTypeStr=boolean
  Switch : Switch  Criteria=u2 > Threshold  OutDataTypeStr=fixdt(0, 4, 0)  SaturateOnIntegerOverflow=off  InputSameDT=off
  data2 : Outport  SampleTime=3.00000003e-08
  valid : Outport  Port=2  SampleTime=3.00000003e-08
  wires:
  Switch/1 -> Add/1
  Logical Operator9/1 -> Logical Operator16/1
  Logical Operator8/1 -> Logical Operator15/1, Logical Operator9/3
  Logical Operator7/1 -> Logical Operator14/1, Logical Operator8/3, Logical Operator9/2
  Logical Operator6/1 -> Logical Operator9/1
  Logical Operator5/1 -> Logical Operator8/1
  Logical Operator4/1 -> Logical Operator7/1
  Logical Operator3/1 -> Logical Operator12/1, Logical Operator2/1, Logical Operator4/1, Logical Operator5/1, Logical Operator6/1
  Logical Operator23/1 -> Switch/2
  Logical Operator22/1 -> Logical Operator23/2
  Logical Operator21/1 -> Logical Operator23/1
  Logical Operator20/1 -> valid/1, Logical Operator22/1
  Logical Operator2/1 -> Logical Operator13/1, Logical Operator6/4, Logical Operator7/2, Logical Operator8/2
  Logical Operator19/1 -> Bit Concat/3, Logical Operator20/4, Logical Operator21/3
  Logical Operator18/1 -> Bit Concat/2, Logical Operator20/3, Logical Operator21/2
  Logical Operator17/1 -> Bit Concat/1, Logical Operator20/1, Logical Operator21/1
  Logical Operator16/1 -> Logical Operator19/3
  Logical Operator15/1 -> Logical Operator18/4
  Logical Operator14/1 -> Logical Operator18/3, Logical Operator19/4
  Logical Operator13/1 -> Logical Operator17/4
  Logical Operator12/1 -> Logical Operator17/3, Logical Operator19/2
  Logical Operator11/1 -> Logical Operator17/2, Logical Operator18/2
  Logical Operator10/1 -> Logical Operator17/1, Logical Operator18/1, Logical Operator19/1
  Logical Operator1/1 -> Logical Operator11/1, Logical Operator2/2, Logical Operator3/1, Logical Operator4/2, Logical Operator5/2, Logical Operator6/2
  Logical Operator/1 -> Logical Operator1/1, Logical Operator10/1, Logical Operator2/3, Logical Operator3/2, Logical Operator4/3, Logical Operator5/3, Logical Operator6/3
  Constant3/1 -> Switch/1
  Constant2/1 -> Switch/3
  Bit Concat/1 -> Add/2
  Add/1 -> data2/1
  D0/1 -> Logical Operator20/2
  D1/1 -> Logical Operator9/4
  D2/1 -> Logical Operator8/4
  D3/1 -> Logical Operator7/3
  D4/1 -> Logical Operator2/4
  D5/1 -> Logical Operator3/3
  D6/1 -> Logical Operator1/2
  D7/1 -> Logical Operator/1
